simulink model "block"  (Simulink 7.9)
settings: Solver=ode45  StartTime=0.0  StopTime=8.0  RelTol=1e-3
settings Model: Creator=Nick  LastModifiedBy=Nick

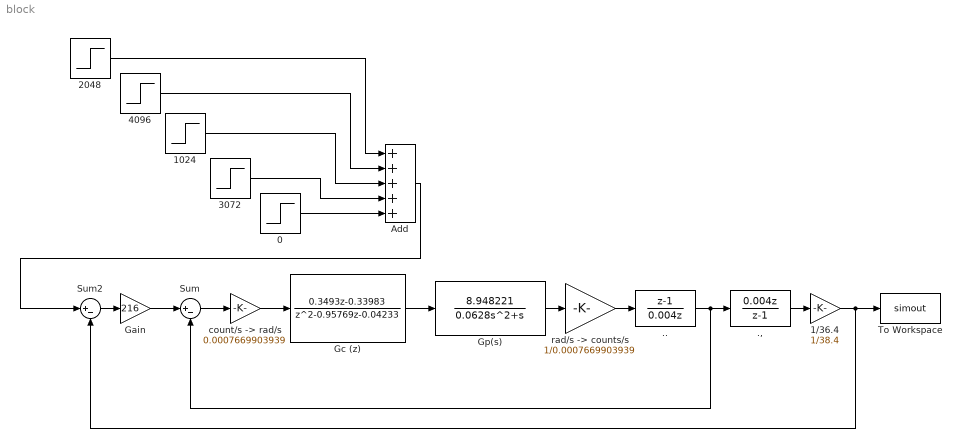
== system block ==
  ., : DiscreteTransferFcn  Numerator=[0.004 0]  Denominator=[1 -1]
  .. : DiscreteTransferFcn  Numerator=[1 -1]  Denominator=[0.004 0]  SampleTime=0.004
  0 : Step  Time=6.4  After=-30720  SampleTime=0.004
  1/36.4 : Gain  Gain=1/38.4  SampleTime=0.004
  1024 : Step  Time=3.2  After=10240*4  SampleTime=0.004
  2048 : Step  Time=0  After=10240*6  SampleTime=0.004
  3072 : Step  Time=4.8  After=10240*-5  SampleTime=0.004
  4096 : Step  Time=1.6  After=-10240*2  SampleTime=0.004
  Add : Sum  Inputs=+++++
  Gain : Gain  Gain=216  SampleTime=0.004
  Gc (z) : DiscreteTransferFcn  Tag=z  Numerator=[0.3493 -0.33983]  Denominator=[1 -0.95769 -0.04233]  SampleTime=0.004
  Gp(s) : TransferFcn  Numerator=[8.948221]  Denominator=[0.0628 1 0]
  Sum : Sum  Inputs=|+-  SampleTime=0.004
  Sum2 : Sum  Inputs=|+-  SampleTime=0.004
  To Workspace : ToWorkspace  VariableName=simout  SampleTime=0.004
  "count/s -> rad/s" : Gain  Gain=0.0007669903939  SampleTime=0.004
  "rad/s -> counts/s" : Gain  Gain=1/0.0007669903939  SampleTime=0.004
  wires:
  Gain/1 -> Sum/1
  Sum2/1 -> Gain/1
  Sum/1 -> "count/s -> rad/s"/1
  "count/s -> rad/s"/1 -> Gc (z)/1
  Gc (z)/1 -> Gp(s)/1
  Gp(s)/1 -> "rad/s -> counts/s"/1
  "rad/s -> counts/s"/1 -> ../1
  ../1 -> .,/1, Sum/2
  .,/1 -> 1/36.4/1
  1/36.4/1 -> To Workspace/1, Sum2/2
  Add/1 -> Sum2/1
  2048/1 -> Add/1
  4096/1 -> Add/2
  1024/1 -> Add/3
  3072/1 -> Add/4
  0/1 -> Add/5
